simulink model "Demo919"  (R2018b)
settings: Solver=ode3  StartTime=0.0  StopTime=10  FixedStep=0.0005  RelTol=1e-3  EnableMultiTasking=on
values from neighbouring files (symbols this model uses):
  ADS1 = [1000 4000]    [data_new1.m]
  ADS2 = [900 4100]    [data_new1.m]
  br_opening = [0 20 40 60 80 100]    [data_new1.m]
  BRAKE = [485 1288 2091 2894 3697 4500]    [data_new1.m]
  InerWheel_Angle = [0 0.001 0.502 1.006 1.514 2.024 2.538 3.055 3.575 4.098 4.625 5.155 5.689 6.226 6.767 7.311 7.859 8.411 8.967 9.527 10.091 10.659 11.231 11.807 12.387 12.972 13.561 14.154 14.752 15.354 15.961 16.572 17.187 17.807 18.432 19.062 19.696 20.334 20.977 21.625 22.277 22.934 23.596 24.262 24.932 25.607 26.286 26.970 27.657 28.349 29.045 29.745 30.448 31.155 31.866]    [data_new1.m]
  OuterWheel_Angle = [0 0.001 0.501 1.001 1.501 2.001 2.501	3.001 3.501	4.001 4.501	5.001 5.501	6.001 6.501	7.001 7.501	8.001 8.501	9.001 9.501	10.001 10.501 11.001 11.501 12.001 12.501 13.001 13.501	14.001 14.501 15.001 15.501 16.001 16.501 17.001 17.501 18.001 18.501 19.001 19.501	20.001 20.501 21.001 21.501	22.001 22.501 23.001 23.501	24.001 24.501 25.001 25.501 26.001 26.501]    [data_new1.m]
  PUMP = [0 1000 2000 3000 4000 5000]    [data_new1.m]
  SteeringAngle_Cal = [-90 0 90]    [data_new1.m]
  SteeringAngle_Sensor = [640 1840 3041]    [data_new1.m]
  th_opening = [0 100]    [data_new1.m]
undefined symbols (not defined in the file or in its folder): D, I_AN06_5V, I_AN08_5V, I_AN09_5V, I_AN10_5V, I_HALL1, I_HALL2, I_SW01_L, I_SW10_L, I_SW11_H, I_SW12_H, I_SW13_H, I_SW14_H, I_SW15_H, I_SW16_H, I_SW17_H, I_SW18_H, I_SW19_H, I_SW20_H, O_PWM1_LS0A7, O_PWM2_LS0A7, O_SW02_LS0A4, O_SW13_HS1A, O_SW14_HS1A
libraries: ec5744lib x137, simulink x20, canmsglib x11
(part 1 of 5)
settings Model: Creator=30855  LastModifiedBy=Lenovo
settings OptimizationCC: DefaultParameterBehavior=Inlined  InlineInvariantSignals=on  EnhancedBackFolding=on  ExpressionFolding=off  PassReuseOutputArgsAs=Individual arguments  RollThreshold=65  StateBitsets=on  DataBitsets=on  ZeroExternalMemoryAtStartup=off  ZeroInternalMemoryAtStartup=off  EfficientFloat2IntCast=on  OptimizeBlockOrder=speed  DifferentSizesBufferReuse=on
settings DebuggingCC: InheritedTsInSrcMsg=none  ParameterTunabilityLossMsg=error
settings HardwareCC: ProdBitPerPointer=32  ProdBitPerSizeT=32  ProdBitPerPtrDiffT=32  ProdLargestAtomicInteger=Long  ProdLargestAtomicFloat=Double  ProdEndianess=BigEndian  ProdWordSize=32  ProdHWDeviceType=Freescale MPC5500
settings SFSimCC: MATLABDynamicMemAlloc=off
settings RTWCC: SystemTargetFile=ec5744.tlc  MakeCommand=make_rtw optimized_fixed_point=1  GenerateMakefile=off  TemplateMakefile=ec5744_lcc.tmf  PostCodeGenCommand=ec5744_pst_s2(buildInfo)  Description=Target for EC5744  GenerateReport=on  IncludeHyperlinkInReport=on  LaunchReport=on  GenerateTraceInfo=on  GenerateTraceReport=on  GenerateTraceReportSl=on  GenerateTraceReportSf=on  GenerateTraceReportEml=on
settings CodeAppCC: ForceParamTrailComments=on  IgnoreCustomStorageClasses=off  OperatorAnnotations=on  SimulinkDataObjDesc=on  SFDataObjDesc=on  InsertBlockDesc=on
settings STFCustomTargetCC: TargetLangStandard=C99 (ISO)  MultiwordLength=256  ModelReferenceCompliant=off  IncludeMdlTerminateFcn=off  CombineOutputUpdateFcns=on  SuppressErrorStatus=on  ERTCustomFileBanners=on  SupportContinuousTime=off  SupportNonInlinedSFcns=off  RemoveResetFunc=on  MATLABClassNameForMDSCustomization=Simulink.SoftwareTarget.ERTCustomization  SystemTargetFile=ec5744.tlc
settings ERTTargetCC: TargetLangStandard=C99 (ISO)  ModelReferenceCompliant=off  ParMdlRefBuildCompliant=off  CompOptLevelCompliant=off  ConcurrentExecutionCompliant=off  IncludeMdlTerminateFcn=off  SuppressErrorStatus=on  ModelStepFunctionPrototypeControlCompliant=off  CPPClassGenCompliant=off  UseToolchainInfoCompliant=off  GenerateASAP2=on  InlinedParameterPlacement=NonHierarchical  ERTSrcFileBannerTemplate=ec5744_code_template.cgt  ERTHdrFileBannerTemplate=ec5744_code_template.cgt  ERTDataSrcFileTemplate=ec5744_code_template.cgt  ERTDataHdrFileTemplate=ec5744_code_template.cgt  ERTCustomFileTemplate=ec5744_file_process.tlc

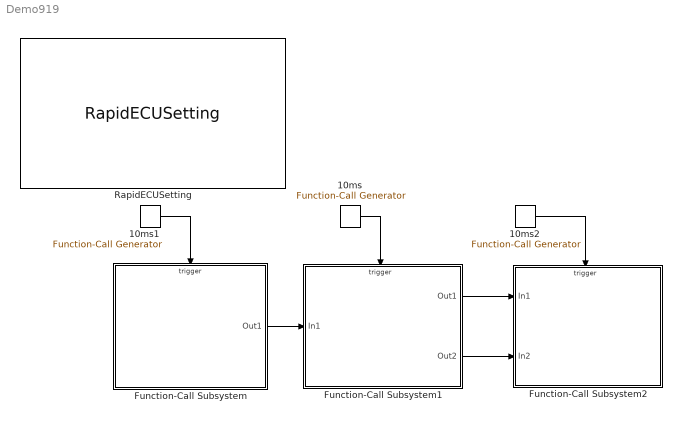
== system Demo919 ==
  10ms : simulink/Ports & Subsystems/Function-Call Generator  sample_time=0.01  numberOfIterations=1
  10ms1 : simulink/Ports & Subsystems/Function-Call Generator  sample_time=0.01  numberOfIterations=1
  10ms2 : simulink/Ports & Subsystems/Function-Call Generator  sample_time=0.01  numberOfIterations=1
  Function-Call Subsystem : Subsystem  TreatAsAtomicUnit=on
  Function-Call Subsystem1 : Subsystem  TreatAsAtomicUnit=on
  Function-Call Subsystem2 : Subsystem  TreatAsAtomicUnit=on
  RapidECUSetting : ec5744lib/RapidECU_U3/RapidECUSetting
      link override CAN: apdf=9  acmt=Extended(29-bit ID)  bpdf=9  cpdf=4  aboi=off  bcmt=Standard(11-bit ID)
      link override LIN: abrt=19200
      settings: SourceProductName=ECUCoder for MPC5744
  wires:
  10ms/1 -> Function-Call Subsystem1/Trigger
  Function-Call Subsystem/1(Out1) -> Function-Call Subsystem1/1(In1)
  Function-Call Subsystem1/1(Out1) -> Function-Call Subsystem2/1(In1)
  Function-Call Subsystem1/2(Out2) -> Function-Call Subsystem2/2(In2)
  10ms1/1 -> Function-Call Subsystem/Trigger
  10ms2/1 -> Function-Call Subsystem2/Trigger

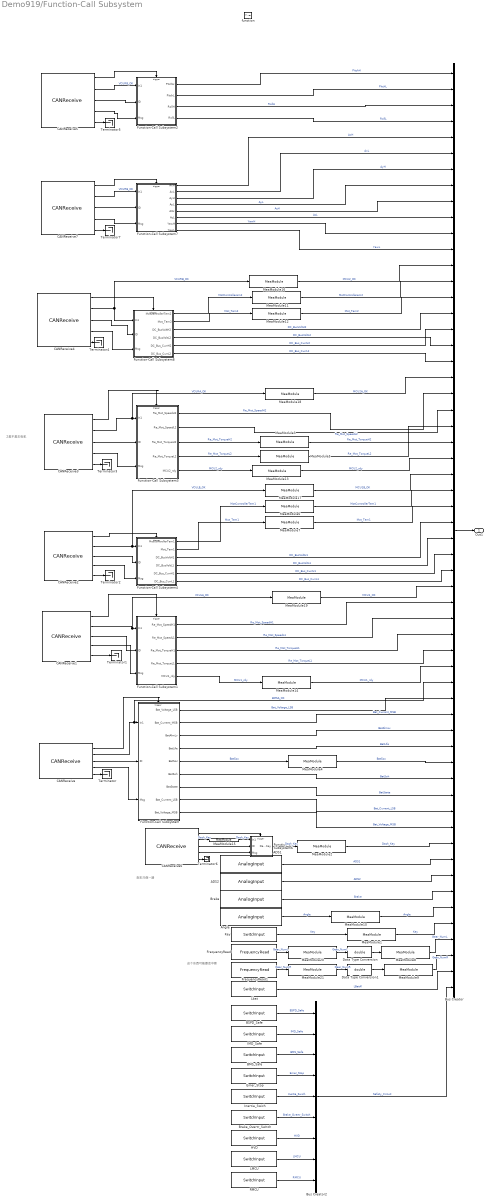
== system Demo919/Function-Call Subsystem ==
  note: 2是不是左电机
  note: 这个东西可能要走中断
  note: 刹车只做一路
  function : TriggerPort  TriggerType=function-call  VariantControl=Variant
  ADS1 : ec5744lib/RapidECU_U3/01BasicInput/AnalogInput  channel=54:I_AN08_5V  sampletime=-1
      settings: SourceProductName=ECUCoder for MPC5744
  ADS2 : ec5744lib/RapidECU_U3/01BasicInput/AnalogInput  channel=55:I_AN09_5V  sampletime=-1
      settings: SourceProductName=ECUCoder for MPC5744
  Angle : ec5744lib/RapidECU_U3/01BasicInput/AnalogInput  channel=56:I_AN10_5V  sampletime=-1
      settings: SourceProductName=ECUCoder for MPC5744
  BMS_Safe : ec5744lib/RapidECU_U3/01BasicInput/SwitchInput  channel=100:I_SW14_H  sampletime=-1
      settings: SourceProductName=ECUCoder for MPC5744
  BSPD_Safe : ec5744lib/RapidECU_U3/01BasicInput/SwitchInput  channel=46:I_SW12_H  sampletime=-1
      settings: SourceProductName=ECUCoder for MPC5744
  Brake : ec5744lib/RapidECU_U3/01BasicInput/AnalogInput  channel=52:I_AN06_5V  sampletime=-1
      settings: SourceProductName=ECUCoder for MPC5744
  Brake_Overtr_Switch : ec5744lib/RapidECU_U3/01BasicInput/SwitchInput  channel=104:I_SW17_H  sampletime=-1
      settings: SourceProductName=ECUCoder for MPC5744
  Bus Creator : BusCreator  Inputs=58
  Bus Creator2 : BusCreator  Inputs=9
  CANReceive : ec5744lib/RapidECU_U3/04CANCommunication/CANReceive  canmodule=0  canbuffer=16  canmessageid=hex2dec('186040F3')  canmessagetype=Extended(29-bit ID)  datalength=8  sampletime=-1
      settings: SourceProductName=ECUCoder for MPC5744
  CANReceive1 : ec5744lib/RapidECU_U3/04CANCommunication/CANReceive  canmodule=0  canbuffer=6  canmessageid=hex2dec('CFFC6EF')  canmessagetype=Extended(29-bit ID)  datalength=8  sampletime=-1
      settings: SourceProductName=ECUCoder for MPC5744
  CANReceive2 : ec5744lib/RapidECU_U3/04CANCommunication/CANReceive  canmodule=0  canbuffer=4  canmessageid=hex2dec('CFFC7EF')  canmessagetype=Extended(29-bit ID)  datalength=8  sampletime=-1
      settings: SourceProductName=ECUCoder for MPC5744
  CANReceive3 : ec5744lib/RapidECU_U3/04CANCommunication/CANReceive  canmodule=0  canbuffer=2  canmessageid=hex2dec('CB221EF')  canmessagetype=Extended(29-bit ID)  datalength=8  sampletime=-1
      settings: SourceProductName=ECUCoder for MPC5744
  CANReceive4 : ec5744lib/RapidECU_U3/04CANCommunication/CANReceive  canmodule=0  canbuffer=0  canmessageid=hex2dec('CB321EF')  canmessagetype=Extended(29-bit ID)  datalength=8  sampletime=-1
      settings: SourceProductName=ECUCoder for MPC5744
  CANReceive5 : ec5744lib/RapidECU_U3/04CANCommunication/CANReceive  canmodule=1  canbuffer=0  canmessageid=hex2dec('157')  canmessagetype=Standard(11-bit ID)  datalength=8  sampletime=-1
      settings: SourceProductName=ECUCoder for MPC5744
  CANReceive6 : ec5744lib/RapidECU_U3/04CANCommunication/CANReceive  canmodule=1  canbuffer=5  canmessageid=hex2dec('155')  canmessagetype=Standard(11-bit ID)  datalength=8  sampletime=-1
      settings: SourceProductName=ECUCoder for MPC5744
  CANReceive7 : ec5744lib/RapidECU_U3/04CANCommunication/CANReceive  canmodule=1  canbuffer=0  canmessageid=hex2dec('156')  canmessagetype=Standard(11-bit ID)  datalength=8  sampletime=-1
      settings: SourceProductName=ECUCoder for MPC5744
  Data Type Conversion : DataTypeConversion  OutDataTypeStr=double
  Data Type Conversion1 : DataTypeConversion  OutDataTypeStr=double
  Emer_Stop : ec5744lib/RapidECU_U3/01BasicInput/SwitchInput  channel=102:I_SW15_H  sampletime=-1
      settings: SourceProductName=ECUCoder for MPC5744
  FrequencyRead : ec5744lib/RapidECU_U3/01BasicInput/FrequencyRead  channel=37:I_HALL1  sampletime=-1
      settings: SourceProductName=ECUCoder for MPC5744
  FrequencyRead1 : ec5744lib/RapidECU_U3/01BasicInput/FrequencyRead  channel=103:I_SW16_H/I_HALL2  sampletime=-1
      settings: SourceProductName=ECUCoder for MPC5744
  Function-Call Subsystem : Subsystem  TreatAsAtomicUnit=on
  Function-Call Subsystem1 : Subsystem  TreatAsAtomicUnit=on
  Function-Call Subsystem2 : Subsystem  TreatAsAtomicUnit=on
  Function-Call Subsystem3 : Subsystem  TreatAsAtomicUnit=on
  Function-Call Subsystem4 : Subsystem  TreatAsAtomicUnit=on
  Function-Call Subsystem6 : Subsystem  TreatAsAtomicUnit=on
  Function-Call Subsystem7 : Subsystem  TreatAsAtomicUnit=on
  Function-Call Subsystem8 : Subsystem  TreatAsAtomicUnit=on
  HVD : ec5744lib/RapidECU_U3/01BasicInput/SwitchInput  channel=105:I_SW18_H  sampletime=-1
      settings: SourceProductName=ECUCoder for MPC5744
  IMD_Safe : ec5744lib/RapidECU_U3/01BasicInput/SwitchInput  channel=65:I_SW13_H  sampletime=-1
      settings: SourceProductName=ECUCoder for MPC5744
  Inertia_Swich : ec5744lib/RapidECU_U3/01BasicInput/SwitchInput  channel=44:I_SW11_H  sampletime=-1
      settings: SourceProductName=ECUCoder for MPC5744
  Key : ec5744lib/RapidECU_U3/01BasicInput/SwitchInput  channel=29:I_SW10_L  sampletime=-1
      settings: SourceProductName=ECUCoder for MPC5744
  LMCU : ec5744lib/RapidECU_U3/01BasicInput/SwitchInput  channel=112:I_SW19_H  sampletime=-1
      settings: SourceProductName=ECUCoder for MPC5744
  Lbat : ec5744lib/RapidECU_U3/01BasicInput/SwitchInput  channel=6:I_SW01_L  sampletime=-1
      settings: SourceProductName=ECUCoder for MPC5744
  MeaModule1 : ec5744lib/RapidECU_U3/07Calibration/MeaModule  signal=Key
      settings: SourceProductName=ECUCoder for MPC5744
  MeaModule10 : ec5744lib/RapidECU_U3/07Calibration/MeaModule  signal=Angle
      settings: SourceProductName=ECUCoder for MPC5744
  MeaModule11 : ec5744lib/RapidECU_U3/07Calibration/MeaModule  signal=MotConTem2
      settings: SourceProductName=ECUCoder for MPC5744
  MeaModule12 : ec5744lib/RapidECU_U3/07Calibration/MeaModule  signal=MotTem2
      settings: SourceProductName=ECUCoder for MPC5744
  MeaModule13 : ec5744lib/RapidECU_U3/07Calibration/MeaModule  signal=MCU2_rdy
      settings: SourceProductName=ECUCoder for MPC5744
  MeaModule14 : ec5744lib/RapidECU_U3/07Calibration/MeaModule  signal=MCU1_rdy
      settings: SourceProductName=ECUCoder for MPC5744
  MeaModule15 : ec5744lib/RapidECU_U3/07Calibration/MeaModule  signal=CANOK
      settings: SourceProductName=ECUCoder for MPC5744
  MeaModule16 : ec5744lib/RapidECU_U3/07Calibration/MeaModule  signal=MCU2B_OK
      settings: SourceProductName=ECUCoder for MPC5744
  MeaModule17 : ec5744lib/RapidECU_U3/07Calibration/MeaModule  signal=MCU1B_OK
      settings: SourceProductName=ECUCoder for MPC5744
  MeaModule18 : ec5744lib/RapidECU_U3/07Calibration/MeaModule  signal=MCU2A_OK
      settings: SourceProductName=ECUCoder for MPC5744
  MeaModule19 : ec5744lib/RapidECU_U3/07Calibration/MeaModule  signal=MCU1A_OK
      settings: SourceProductName=ECUCoder for MPC5744
  MeaModule2 : ec5744lib/RapidECU_U3/07Calibration/MeaModule  signal=Dash_KEY
      settings: SourceProductName=ECUCoder for MPC5744
  MeaModule20 : ec5744lib/RapidECU_U3/07Calibration/MeaModule  signal=HALL_l
      settings: SourceProductName=ECUCoder for MPC5744
  MeaModule21 : ec5744lib/RapidECU_U3/07Calibration/MeaModule  signal=HALL_r
      settings: SourceProductName=ECUCoder for MPC5744
  MeaModule3 : ec5744lib/RapidECU_U3/07Calibration/MeaModule  signal=Re_Mot_ToqH
      settings: SourceProductName=ECUCoder for MPC5744
  MeaModule4 : ec5744lib/RapidECU_U3/07Calibration/MeaModule  signal=BatSoc
      settings: SourceProductName=ECUCoder for MPC5744
  MeaModule5 : ec5744lib/RapidECU_U3/07Calibration/MeaModule  signal=Re_MotToqL
      settings: SourceProductName=ECUCoder for MPC5744
  MeaModule6 : ec5744lib/RapidECU_U3/07Calibration/MeaModule  signal=MotConTem1
      settings: SourceProductName=ECUCoder for MPC5744
  MeaModule7 : ec5744lib/RapidECU_U3/07Calibration/MeaModule  signal=MotTem1
      settings: SourceProductName=ECUCoder for MPC5744
  MeaModule8 : ec5744lib/RapidECU_U3/07Calibration/MeaModule  signal=HALL_L
      settings: SourceProductName=ECUCoder for MPC5744
  MeaModule9 : ec5744lib/RapidECU_U3/07Calibration/MeaModule  signal=HALL_R
      settings: SourceProductName=ECUCoder for MPC5744
  RMCU : ec5744lib/RapidECU_U3/01BasicInput/SwitchInput  channel=113:I_SW20_H  sampletime=-1
      settings: SourceProductName=ECUCoder for MPC5744
  Terminator{,1..7} (8 alike) : Terminator
  Out1 : Outport
  wires:
  ADS1/1 -> Bus Creator/50  "ADS1"
  ADS2/1 -> Bus Creator/51  "ADS2"
  Brake/1 -> Bus Creator/52  "Brake"
  Angle/1 -> MeaModule10/1  "Angle"
  Bus Creator/1 -> Out1/1
  Key/1 -> MeaModule1/1  "Key"
  CANReceive/1 -> Function-Call Subsystem/Trigger
  CANReceive/2 -> Bus Creator/39, Function-Call Subsystem/1(In1)  "BMSA_OK"
  CANReceive/3 -> Function-Call Subsystem/2(ID)
  CANReceive/4 -> Function-Call Subsystem/3(Msg)
  CANReceive/5 -> Terminator/1
  Function-Call Subsystem/1(Bat_Voltage_LSB) -> Bus Creator/40  "Bat_Voltage_LSB"
  Function-Call Subsystem/2(Bat_Current_MSB) -> Bus Creator/41  "Bat_Current_MSB"
  Function-Call Subsystem/3(BatAlmLv) -> Bus Creator/42  "BatAlmLv"
  Function-Call Subsystem/4(BatLife) -> Bus Creator/43  "BatLife"
  Function-Call Subsystem/5(BatSoc) -> MeaModule4/1  "BatSoc"
  Function-Call Subsystem/6(BatSoh) -> Bus Creator/45  "BatSoh"
  Function-Call Subsystem/7(BatState) -> Bus Creator/46  "BatState"
  Function-Call Subsystem/8(Bat_Current_LSB) -> Bus Creator/47  "Bat_Current_LSB"
  FrequencyRead/1 -> MeaModule20/1  "Gear_NumL"
  CANReceive1/5 -> Terminator1/1
  CANReceive1/4 -> Function-Call Subsystem1/3(Msg)
  CANReceive1/3 -> Function-Call Subsystem1/2(ID)
  CANReceive1/2 -> MeaModule19/1, Function-Call Subsystem1/1(In1)  "VCULA_OK"
  CANReceive1/1 -> Function-Call Subsystem1/Trigger
  CANReceive2/1 -> Function-Call Subsystem4/Trigger
  CANReceive2/2 -> Function-Call Subsystem4/1(In1), MeaModule17/1  "VCULB_OK"
  CANReceive2/3 -> Function-Call Subsystem4/2(ID)
  CANReceive2/4 -> Function-Call Subsystem4/3(Msg)
  CANReceive2/5 -> Terminator2/1
  CANReceive3/5 -> Terminator3/1
  CANReceive3/4 -> Function-Call Subsystem3/3(Msg)
  CANReceive3/3 -> Function-Call Subsystem3/2(ID)
  CANReceive3/2 -> MeaModule18/1, Function-Call Subsystem3/1(In1)  "VCURA_OK"
  CANReceive3/1 -> Function-Call Subsystem3/Trigger
  CANReceive4/1 -> Function-Call Subsystem8/Trigger
  CANReceive4/2 -> Function-Call Subsystem8/1(In1), MeaModule16/1  "VCURB_OK"
  CANReceive4/3 -> Function-Call Subsystem8/2(ID)
  CANReceive4/4 -> Function-Call Subsystem8/3(Msg)
  CANReceive4/5 -> Terminator4/1
  Function-Call Subsystem1/4(Re_Mot_TorqueL1) -> Bus Creator/37  "Re_Mot_TorqueL1"
  Function-Call Subsystem1/3(Re_Mot_TorqueH1) -> Bus Creator/36  "Re_Mot_TorqueH1"
  Function-Call Subsystem1/2(Re_Mot_SpeedL1) -> Bus Creator/35  "Re_Mot_SpeedL1"
  Function-Call Subsystem1/1(Re_Mot_SpeedH1) -> Bus Creator/34  "Re_Mot_SpeedH1"
  Function-Call Subsystem4/2(Mot_Tem1) -> MeaModule7/1  "Mot_Tem1"
  Function-Call Subsystem4/1(MotControllerTem1) -> MeaModule6/1  "MotControllerTem1"
  Function-Call Subsystem3/4(Re_Mot_TorqueL2) -> MeaModule5/1  "Re_Mot_TorqueL2"
  Function-Call Subsystem3/3(Re_Mot_TorqueH2) -> MeaModule3/1  "Re_Mot_TorqueH2"
  Function-Call Subsystem3/2(Re_Mot_SpeedL2) -> Bus Creator/22  "Re_Mot_SpeedL2"
  Function-Call Subsystem3/1(Re_Mot_SpeedH2) -> Bus Creator/21  "Re_Mot_SpeedH2"
  Function-Call Subsystem8/2(Mot_Tem2) -> MeaModule12/1  "Mot_Tem2"
  Function-Call Subsystem8/1(MotControllerTem2) -> MeaModule11/1  "MotControllerem2"
  Function-Call Subsystem/9(Bat_Voltage_MSB) -> Bus Creator/48  "Bat_Voltage_MSB"
  FrequencyRead1/1 -> MeaModule21/1  "Gear_NumR"
  CANReceive6/1 -> Function-Call Subsystem6/Trigger
  CANReceive6/3 -> Function-Call Subsystem6/2(ID)
  CANReceive6/4 -> Function-Call Subsystem6/3(Msg)
  CANReceive6/5 -> Terminator6/1
  Function-Call Subsystem6/1(Dash_Key) -> MeaModule2/1  "Dash_Key"
  MeaModule1/1 -> Bus Creator/54  "Key"
  MeaModule3/1 -> Bus Creator/23  "Re_Mot_TorqueH2"
  MeaModule5/1 -> Bus Creator/24  "Re_Mot_TorqueL2"
  MeaModule6/1 -> Bus Creator/27  "MotControllerTem1"
  MeaModule7/1 -> Bus Creator/28  "Mot_Tem1"
  MeaModule8/1 -> Bus Creator/55  "Gear_NumL"
  MeaModule9/1 -> Bus Creator/56  "Gear_NumR"
  MeaModule11/1 -> Bus Creator/14  "MotControllerem2"
  MeaModule12/1 -> Bus Creator/15  "Mot_Tem2"
  MeaModule2/1 -> Bus Creator/49  "Dash_Key"
  CANReceive6/2 -> MeaModule15/1  "Dash_Key"
  Function-Call Subsystem4/3(DC_BusVoltH1) -> Bus Creator/29  "DC_BusVoltH1"
  Function-Call Subsystem8/3(DC_BusVoltH2) -> Bus Creator/16  "DC_BusVoltH2"
  Function-Call Subsystem8/6("DC_Bus_CurrL2 ") -> Bus Creator/19  "DC_Bus_CurrL2"
  Function-Call Subsystem4/4(DC_BusVoltL1) -> Bus Creator/30  "DC_BusVoltL1"
  MeaModule4/1 -> Bus Creator/44  "BatSoc"
  Function-Call Subsystem1/5(MCU1_rdy) -> MeaModule14/1  "MCU1_rdy"
  Function-Call Subsystem3/5(MCU2_rdy) -> MeaModule13/1  "MCU2_rdy"
  Data Type Conversion/1 -> MeaModule8/1
  Data Type Conversion1/1 -> MeaModule9/1
  CANReceive7/1 -> Function-Call Subsystem7/Trigger
  CANReceive7/3 -> Function-Call Subsystem7/2(ID)
  CANReceive7/4 -> Function-Call Subsystem7/3(Msg)
  CANReceive7/2 -> Function-Call Subsystem7/1(In1)  "VCURB_OK"
  CANReceive7/5 -> Terminator7/1
  Function-Call Subsystem7/1(AxH) -> Bus Creator/5  "AxH"
  Function-Call Subsystem7/8(YawL) -> Bus Creator/12  "YawL"
  Function-Call Subsystem7/7(YawH) -> Bus Creator/11  "YawH"
  Function-Call Subsystem7/6(AzL) -> Bus Creator/10  "AzL"
  Function-Call Subsystem7/5(AzH) -> Bus Creator/9  "AzH"
  Function-Call Subsystem7/4(AyL) -> Bus Creator/8  "AyL"
  Function-Call Subsystem7/3(AyH) -> Bus Creator/7  "AyH"
  MeaModule10/1 -> Bus Creator/53  "Angle"
  MeaModule13/1 -> Bus Creator/25  "MCU2_rdy"
  MeaModule14/1 -> Bus Creator/38  "MCU1_rdy"
  Function-Call Subsystem7/2(AxL) -> Bus Creator/6  "AxL"
  MeaModule15/1 -> Function-Call Subsystem6/1(In1)  "Dash_Key"
  Function-Call Subsystem8/4(DC_BusVoltL2) -> Bus Creator/18  "DC_BusVoltL2"
  Function-Call Subsystem8/5(DC_Bus_CurrH2) -> Bus Creator/17  "DC_Bus_CurrH2"
  Function-Call Subsystem4/5(DC_Bus_CurrH1) -> Bus Creator/31  "DC_Bus_CurrH1"
  Function-Call Subsystem4/6(DC_Bus_CurrL1) -> Bus Creator/32  "DC_Bus_CurrL1"
  MeaModule16/1 -> Bus Creator/13  "MCU2_OK"
  MeaModule18/1 -> Bus Creator/20  "MCU2A_OK"
  MeaModule17/1 -> Bus Creator/26  "MCU1B_OK"
  MeaModule19/1 -> Bus Creator/33  "MCU1_OK"
  CANReceive5/2 -> Function-Call Subsystem2/1(In1)  "VCURB_OK"
  CANReceive5/4 -> Function-Call Subsystem2/3(Msg)
  CANReceive5/3 -> Function-Call Subsystem2/2(ID)
  CANReceive5/5 -> Terminator5/1
  CANReceive5/1 -> Function-Call Subsystem2/Trigger
  Function-Call Subsystem2/1(PitchH) -> Bus Creator/1  "PitchH"
  Function-Call Subsystem2/2(PitchL) -> Bus Creator/2  "PitchL"
  Function-Call Subsystem2/3(RollH) -> Bus Creator/3  "RollH"
  Function-Call Subsystem2/4(RollL) -> Bus Creator/4  "RollL"
  Lbat/1 -> Bus Creator/57  "LBatAl"
  Bus Creator2/1 -> Bus Creator/58  "Safety_Circuit"
  HVD/1 -> Bus Creator2/7  "HVD"
  Inertia_Swich/1 -> Bus Creator2/5  "Inertia_Swich"
  BSPD_Safe/1 -> Bus Creator2/1  "BSPD_Safe"
  RMCU/1 -> Bus Creator2/9  "RMCU"
  Emer_Stop/1 -> Bus Creator2/4  "Emer_Stop"
  Brake_Overtr_Switch/1 -> Bus Creator2/6  "Brake_Overtr_Switch"
  LMCU/1 -> Bus Creator2/8  "LMCU"
  BMS_Safe/1 -> Bus Creator2/3  "BMS_Safe"
  IMD_Safe/1 -> Bus Creator2/2  "IMD_Safe"
  MeaModule20/1 -> Data Type Conversion/1  "Gear_NumL"
  MeaModule21/1 -> Data Type Conversion1/1  "Gear_NumR"

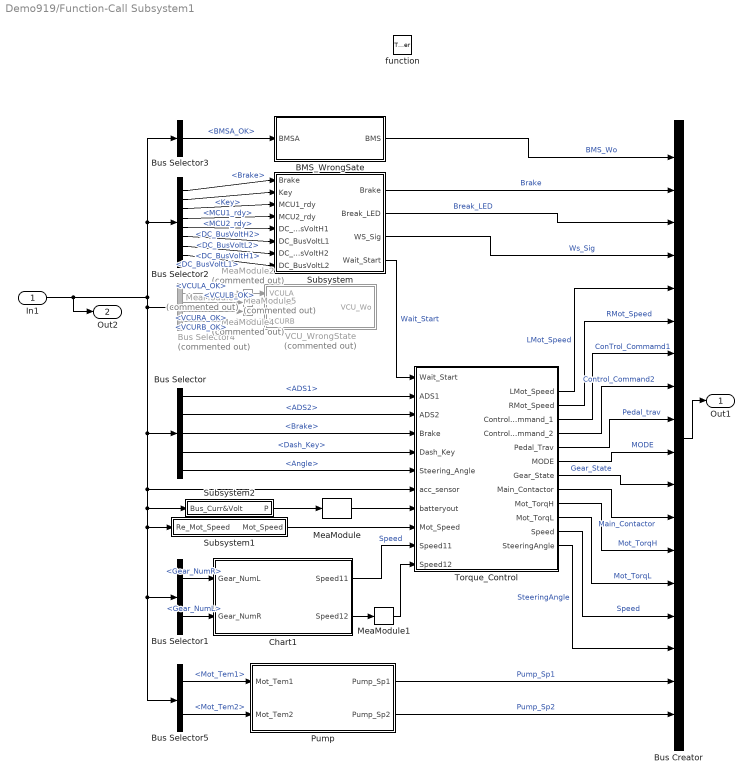
== system Demo919/Function-Call Subsystem1 ==
  In1 : Inport
  "  function" : TriggerPort  TriggerType=function-call  VariantControl=Variant
  BMS_WrongSate : Stateflow chart  TreatAsAtomicUnit=on
  Bus Creator : BusCreator  Inputs=18
  Bus Selector : BusSelector  OutputSignals=ADS1,ADS2,Brake,Dash_Key,Angle
  Bus Selector1 : BusSelector  OutputSignals=Gear_NumR,Gear_NumL
  Bus Selector2 : BusSelector  OutputSignals=Brake,Key,MCU1_rdy,MCU2_rdy,DC_BusVoltH2,DC_BusVoltL2,DC_BusVoltH1,DC_BusVoltL1
  Bus Selector3 : BusSelector  OutputSignals=BMSA_OK
  Bus Selector4 : BusSelector  Commented=on  OutputSignals=VCULA_OK,VCULB_OK,VCURA_OK,VCURB_OK
  Bus Selector5 : BusSelector  OutputSignals=Mot_Tem1,Mot_Tem2
  Chart1 : Stateflow chart  TreatAsAtomicUnit=on
  MeaModule : ec5744lib/RapidECU_U3/07Calibration/MeaModule  signal=P
      settings: SourceProductName=ECUCoder for MPC5744
  MeaModule1 : ec5744lib/RapidECU_U3/07Calibration/MeaModule  signal=S12
      settings: SourceProductName=ECUCoder for MPC5744
  MeaModule2 : ec5744lib/RapidECU_U3/07Calibration/MeaModule  Commented=on  signal=VCULA
      settings: SourceProductName=ECUCoder for MPC5744
  MeaModule3 : ec5744lib/RapidECU_U3/07Calibration/MeaModule  Commented=on  signal=VCUlb
      settings: SourceProductName=ECUCoder for MPC5744
  MeaModule4 : ec5744lib/RapidECU_U3/07Calibration/MeaModule  Commented=on  signal=VCUra
      settings: SourceProductName=ECUCoder for MPC5744
  MeaModule5 : ec5744lib/RapidECU_U3/07Calibration/MeaModule  Commented=on  signal=VCUrb
      settings: SourceProductName=ECUCoder for MPC5744
  Pump : Subsystem
  Subsystem : Subsystem
  Subsystem1 : Subsystem
  Subsystem2 : Subsystem
  Torque_Control : Subsystem
  VCU_WrongState : Stateflow chart  Commented=on  TreatAsAtomicUnit=on
  Out1 : Outport
  Out2 : Outport  Port=2
  wires:
  Bus Selector/1 -> Torque_Control/2(ADS1)  "<ADS1>"
  Bus Selector/2 -> Torque_Control/3(ADS2)  "<ADS2>"
  Torque_Control/1(LMot_Speed) -> Bus Creator/5  "LMot_Speed"
  Torque_Control/2(RMot_Speed) -> Bus Creator/6  "RMot_Speed"
  Bus Creator/1 -> Out1/1
  Bus Selector2/2 -> Subsystem/2(Key)  "<Key>"
  Subsystem/4(Wait_Start) -> Torque_Control/1(Wait_Start)  "Wait_Start"
  BMS_WrongSate/1(BMS) -> Bus Creator/1  "BMS_Wo"
  Torque_Control/3("Control_Command_1 ") -> Bus Creator/7  "ConTrol_Commamd1"
  Torque_Control/4(Control_Command_2) -> Bus Creator/8  "Control_Command2"
  Bus Selector2/1 -> Subsystem/1(Brake)  "<Brake>"
  Torque_Control/5(Pedal_Trav) -> Bus Creator/9  "Pedal_trav"
  Bus Selector/4 -> Torque_Control/5("Dash_Key ")  "<Dash_Key>"
  Bus Selector5/1 -> Pump/1(Mot_Tem1)  "<Mot_Tem1>"
  Bus Selector5/2 -> Pump/2(Mot_Tem2)  "<Mot_Tem2>"
  Pump/1(Pump_Sp1) -> Bus Creator/17  "Pump_Sp1"
  Pump/2(Pump_Sp2) -> Bus Creator/18  "Pump_Sp2"
  Subsystem/2(Break_LED) -> Bus Creator/3  "Break_LED"
  Bus Selector/3 -> Torque_Control/4("Brake ")  "<Brake>"
  Bus Selector3/1 -> BMS_WrongSate/1(BMSA)  "<BMSA_OK>"
  Bus Selector4/1 -> MeaModule2/1  "<VCULA_OK>"
  Bus Selector4/2 -> MeaModule3/1  "<VCULB_OK>"
  Bus Selector4/3 -> MeaModule4/1  "<VCURA_OK>"
  Bus Selector4/4 -> MeaModule5/1  "<VCURB_OK>"
  MeaModule2/1 -> VCU_WrongState/1(VCULA)
  MeaModule3/1 -> VCU_WrongState/2(VCULB)
  MeaModule4/1 -> VCU_WrongState/3(VCURA)
  MeaModule5/1 -> VCU_WrongState/4(VCURB)
  Bus Selector1/2 -> Chart1/2(Gear_NumR)  "<Gear_NumL>"
  Bus Selector1/1 -> Chart1/1(Gear_NumL)  "<Gear_NumR>"
  In1/1 -> Out2/1, Bus Selector4/1, Bus Selector5/1, Bus Selector1/1, Subsystem1/1(Re_Mot_Speed), Subsystem2/1(Bus_Curr&Volt), Torque_Control/7(acc_sensor), Bus Selector/1, Bus Selector3/1, Bus Selector2/1
  Torque_Control/11(Speed) -> Bus Creator/15  "Speed"
  Torque_Control/6(MODE) -> Bus Creator/10  "MODE"
  Subsystem/3(WS_Sig) -> Bus Creator/4  "Ws_Sig"
  Torque_Control/7("Gear_State ") -> Bus Creator/11  "Gear_State"
  Torque_Control/8(Main_Contactor) -> Bus Creator/12  "Main_Contactor"
  Bus Selector2/3 -> Subsystem/3(MCU1_rdy)  "<MCU1_rdy>"
  Bus Selector2/4 -> Subsystem/4(MCU2_rdy)  "<MCU2_rdy>"
  Bus Selector2/5 -> Subsystem/5(DC_BusVoltH1)  "<DC_BusVoltH2>"
  Bus Selector2/6 -> Subsystem/6(DC_BusVoltL1)  "<DC_BusVoltL2>"
  Bus Selector2/7 -> Subsystem/7(DC_BusVoltH2)  "<DC_BusVoltH1>"
  Bus Selector2/8 -> Subsystem/8(DC_BusVoltL2)  "<DC_BusVoltL1>"
  Subsystem/1("Brake ") -> Bus Creator/2  "Brake"
  Bus Selector/5 -> Torque_Control/6(Steering_Angle)  "<Angle>"
  Subsystem2/1(P) -> MeaModule/1
  Subsystem1/1(Mot_Speed) -> Torque_Control/9(Mot_Speed)
  Torque_Control/9(Mot_TorqH) -> Bus Creator/13  "Mot_TorqH"
  Torque_Control/10(Mot_TorqL) -> Bus Creator/14  "Mot_TorqL"
  Chart1/1(Speed11) -> Torque_Control/10(Speed11)  "Speed"
  Chart1/2(Speed12) -> MeaModule1/1
  MeaModule/1 -> Torque_Control/8(batteryout)
  MeaModule1/1 -> Torque_Control/11(Speed12)
  Torque_Control/12(SteeringAngle) -> Bus Creator/16  "SteeringAngle"

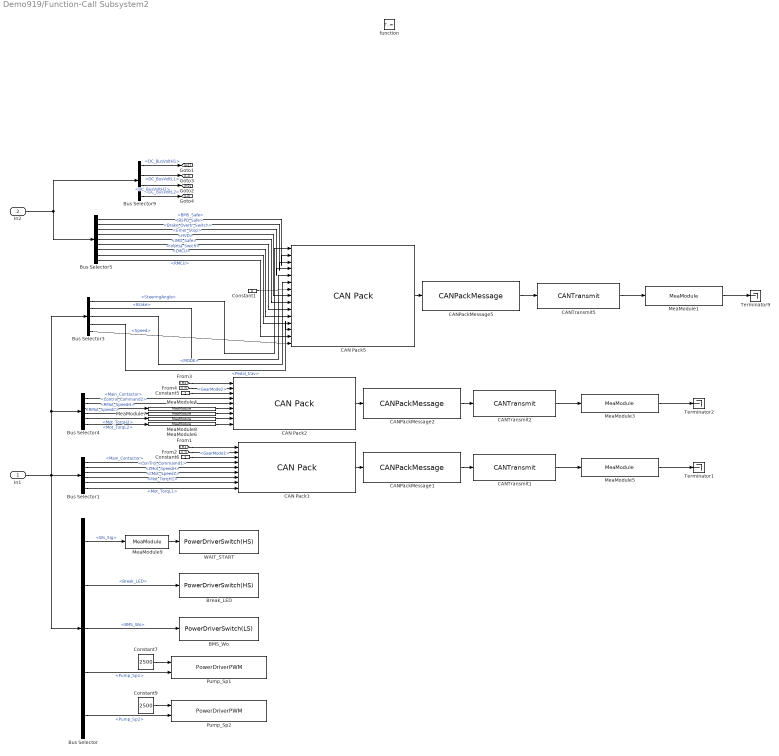
== system Demo919/Function-Call Subsystem2 ==
  In1 : Inport
  In2 : Inport  Port=2
  function : TriggerPort  TriggerType=function-call  VariantControl=Variant
  BMS_Wo : ec5744lib/RapidECU_U3/02PowerDriverSwitch/PowerDriverSwitch(LS)  channel=59:O_SW02_LS0A4  sampletime=-1
      settings: SourceProductName=ECUCoder for MPC5744
  Break_LED : ec5744lib/RapidECU_U3/02PowerDriverSwitch/PowerDriverSwitch(HS)  channel=115:O_SW13_HS1A  sampletime=-1
      settings: SourceProductName=ECUCoder for MPC5744
  Bus Selector : BusSelector  OutputSignals=Ws_Sig,Break_LED,BMS_Wo,Pump_Sp1,Pump_Sp2
  Bus Selector1 : BusSelector  OutputSignals=Main_Contactor,ConTrol_Commamd1,LMot_Speed.LMot_SpeedH,LMot_Speed.LMot_SpeedL,Mot_TorqH.Mot_TorqH1,Mot_TorqL.Mot_TorqL1
  Bus Selector3 : BusSelector  OutputSignals=SteeringAngle,Brake,MODE,Pedal_trav,Speed
  Bus Selector4 : BusSelector  OutputSignals=Main_Contactor,Control_Command2,RMot_Speed.RMot_SpeedH,RMot_Speed.RMot_SpeedL,Mot_TorqH.Mot_TorqH2,Mot_TorqL.Mot_TorqL2
  Bus Selector5 : BusSelector  OutputSignals=Safety_Circuit.BMS_Safe,Safety_Circuit.BSPD_Safe,Safety_Circuit.Brake_Overtr_Switch,Safety_Circuit.Emer_Stop,Safety_Circuit.HVD,Safety_Circuit.IMD_Safe,Safety_Circuit.Inertia_Swich,Safety_Circuit.LMCU,Safety_Circuit.RMCU
  Bus Selector9 : BusSelector  OutputSignals=DC_BusVoltH1,DC_BusVoltL1,DC_BusVoltH2,DC_BusVoltL2
  CAN Pack1 : canmsglib/CAN Pack  CANdbFile=E:\project\DBC_file\MotControl.dbc  MsgList=VCUtoMUC1  MsgName=VCUtoMUC1  MsgIDType=Extended (29-bit identifier)  MsgIdentifier=146927393  MsgLength=8  SignalInfo=DC_Bus_VoltageH1$48$8$1$2$1$0$1$0$0$255$#DC_Bus_VoltageL1$56$8$1$2$1$0$1$0$0$255$#GearState1$40$2$1$2$1$0$1$0$0$3$#Main_contactor1$43$1$1$2$1$0$1$0$0$1$#Tr_ControlMode_Command1$32$8$1$2$1$0$1$0$0$255$#Tr_Mot_SpeedH1$8$8$1$2$1$0$1$0$0$255$#Tr_Mot_SpeedL1$0$8$1$2$1$0$1$0$0$255$#Tr_Mot_TorqH1$24$8$1$2$1$0$1$0$0$255$#Tr_Mot_TorqL1$16$8$1$2$1$0$1$0$0$255$#  NSignals=9  StartBits=str2num('[int32(48);int32(56);int32(40);int32(43);int32(32);int32(8);int32(0);int32(24);int32(16)]')  SignalSizes=str2num('[int32(8);int32(8);int32(2);int32(1);int32(8);int32(8);int32(8);int32(8);int32(8)]')  ByteOrders=str2num('[int32(1);int32(1);int32(1);int32(1);int32(1);int32(1);int32(1);int32(1);int32(1)]')  DataTypes=str2num('[int32(2);int32(2);int32(2);int32(2);int32(2);int32(2);int32(2);int32(2);int32(2)]')  MultiplexTypes=str2num('[int32(1);int32(1);int32(1);int32(1);int32(1);int32(1);int32(1);int32(1);int32(1)]')  MultiplexValues=str2num('[double(0);double(0);double(0);double(0);double(0);double(0);double(0);double(0);double(0)]')  Factors=str2num('[double(1);double(1);double(1);double(1);double(1);double(1);double(1);double(1);double(1)]')  Offsets=str2num('[double(0);double(0);double(0);double(0);double(0);double(0);double(0);double(0);double(0)]')  Minimums=str2num('[double(0);double(0);double(0);double(0);double(0);double(0);double(0);double(0);double(0)]')  Maximums=str2num('[double(255);double(255);double(3);double(1);double(255);double(255);double(255);double(255);double(255)]')  Remote=off  ApplyMinMax=off  BusOutput=off
      settings: SourceProductName=Simulink Real-Time  SourceProductBaseCode=XP  DataFormat=CANdb specified signals
  CAN Pack2 : canmsglib/CAN Pack  CANdbFile=E:\project\DBC_file\MotControl.dbc  MsgList=VCUtoMCU2  MsgName=VCUtoMCU2  MsgIDType=Extended (29-bit identifier)  MsgIdentifier=145878817  MsgLength=8  SignalInfo=DC_Bus_VoltageH2$48$8$1$2$1$0$1$0$0$255$#DC_Bus_VoltrageL2$56$8$1$2$1$0$1$0$0$255$#GearState2$40$2$1$2$1$0$1$0$0$3$#Main_contactor2$43$1$1$2$1$0$1$0$0$1$#Tr_ControlMode_Command2$32$8$1$2$1$0$1$0$0$255$#Tr_Mot_SpeedH2$8$8$1$2$1$0$1$0$0$255$#Tr_Mot_SpeedL2$0$8$1$2$1$0$1$0$0$255$#Tr_Mot_TorqH2$24$8$1$2$1$0$1$0$0$255$#Tr_Mot_TorqL2$16$8$1$2$1$0$1$0$0$255$#  NSignals=9  StartBits=str2num('[int32(48);int32(56);int32(40);int32(43);int32(32);int32(8);int32(0);int32(24);int32(16)]')  SignalSizes=str2num('[int32(8);int32(8);int32(2);int32(1);int32(8);int32(8);int32(8);int32(8);int32(8)]')  ByteOrders=str2num('[int32(1);int32(1);int32(1);int32(1);int32(1);int32(1);int32(1);int32(1);int32(1)]')  DataTypes=str2num('[int32(2);int32(2);int32(2);int32(2);int32(2);int32(2);int32(2);int32(2);int32(2)]')  MultiplexTypes=str2num('[int32(1);int32(1);int32(1);int32(1);int32(1);int32(1);int32(1);int32(1);int32(1)]')  MultiplexValues=str2num('[double(0);double(0);double(0);double(0);double(0);double(0);double(0);double(0);double(0)]')  Factors=str2num('[double(1);double(1);double(1);double(1);double(1);double(1);double(1);double(1);double(1)]')  Offsets=str2num('[double(0);double(0);double(0);double(0);double(0);double(0);double(0);double(0);double(0)]')  Minimums=str2num('[double(0);double(0);double(0);double(0);double(0);double(0);double(0);double(0);double(0)]')  Maximums=str2num('[double(255);double(255);double(3);double(1);double(255);double(255);double(255);double(255);double(255)]')  Remote=off  ApplyMinMax=off  BusOutput=off
      settings: SourceProductName=Simulink Real-Time  SourceProductBaseCode=XP  DataFormat=CANdb specified signals
  CAN Pack5 : canmsglib/CAN Pack  CANdbFile=E:\project\DBC_file\MotControl.dbc  MsgList=VCUtoDash1  MsgName=VCUtoDash1  MsgIDType=Extended (29-bit identifier)  MsgIdentifier=529  MsgLength=8  SignalInfo=Angle$48$8$1$2$1$0$1$0$0$255$#BMS_Safe$33$1$1$2$1$0$1$0$0$1$#BSPD_Safe$40$1$1$2$1$0$1$0$0$1$#Brake_Overtr_Switch$36$1$1$2$1$0$1$0$0$1$#Brake_Val$16$8$1$2$1$0$1$0$0$255$#CarMode$45$3$1$2$1$0$1$0$0$7$#Distance$24$8$1$2$1$0$1$0$0$255$#Emer_Stop$34$1$1$2$1$0$1$0$0$1$#HVD$37$1$1$2$1$0$1$0$0$1$#IMD_Safe$32$1$1$2$1$0$1$0$0$1$#Inertia_Swich$35$1$1$2$1$0$1$0$0$1$#LMCU$38$1$1$2$1$0$1$0$0$1$#Ped_Trav$8$8$1$2$1$0$1$0$0$255$#RMCU$39$1$1$2$1$0$1$0$0$1$#Veh_Sp$0$8$1$2$1$0$1$0$0$255$#  NSignals=15  StartBits=str2num('[int32(48);int32(33);int32(40);int32(36);int32(16);int32(45);int32(24);int32(34);int32(37);int32(32);int32(35);int32(38);int32(8);int32(39);int32(0)]')  SignalSizes=str2num('[int32(8);int32(1);int32(1);int32(1);int32(8);int32(3);int32(8);int32(1);int32(1);int32(1);int32(1);int32(1);int32(8);int32(1);int32(8)]')  ByteOrders=str2num('[int32(1);int32(1);int32(1);int32(1);int32(1);int32(1);int32(1);int32(1);int32(1);int32(1);int32(1);int32(1);int32(1);int32(1);int32(1)]')  DataTypes=str2num('[int32(2);int32(2);int32(2);int32(2);int32(2);int32(2);int32(2);int32(2);int32(2);int32(2);int32(2);int32(2);int32(2);int32(2);int32(2)]')  MultiplexTypes=str2num('[int32(1);int32(1);int32(1);int32(1);int32(1);int32(1);int32(1);int32(1);int32(1);int32(1);int32(1);int32(1);int32(1);int32(1);int32(1)]')  MultiplexValues=str2num('[double(0);double(0);double(0);double(0);double(0);double(0);double(0);double(0);double(0);double(0);double(0);double(0);double(0);double(0);double(0)]')  Factors=str2num('[double(1);double(1);double(1);double(1);double(1);double(1);double(1);double(1);double(1);double(1);double(1);double(1);double(1);double(1);double(1)]')  Offsets=str2num('[double(0);double(0);double(0);double(0);double(0);double(0);double(0);double(0);double(0);double(0);double(0);double(0);double(0);double(0);double(0)]')  Minimums=str2num('[double(0);double(0);double(0);double(0);double(0);double(0);double(0);double(0);double(0);double(0);double(0);double(0);double(0);double(0);double(0)]')  Maximums=str2num('[double(255);double(1);double(1);double(1);double(255);double(7);double(255);double(1);double(1);double(1);double(1);double(1);double(255);double(1);double(255)]')  Remote=off  ApplyMinMax=off  BusOutput=off
      settings: SourceProductName=Simulink Real-Time  SourceProductBaseCode=XP  DataFormat=CANdb specified signals
  CANPackMessage1 : ec5744lib/RapidECU_U3/04CANCommunication/CANPackMessage  datalength=8  sampletime=-1
      settings: SourceProductName=ECUCoder for MPC5744
  CANPackMessage2 : ec5744lib/RapidECU_U3/04CANCommunication/CANPackMessage  datalength=8  sampletime=-1
      settings: SourceProductName=ECUCoder for MPC5744
  CANPackMessage5 : ec5744lib/RapidECU_U3/04CANCommunication/CANPackMessage  datalength=8  sampletime=-1
      settings: SourceProductName=ECUCoder for MPC5744
  CANTransmit1 : ec5744lib/RapidECU_U3/04CANCommunication/CANTransmit  canmodule=0  canbuffer=12  canmessageid=hex2dec('8C1EF21')  canmessagetype=Extended(29-bit ID)  datalength=8  sampletime=-1
      settings: SourceProductName=ECUCoder for MPC5744
  CANTransmit2 : ec5744lib/RapidECU_U3/04CANCommunication/CANTransmit  canmodule=0  canbuffer=10  canmessageid=hex2dec('8B1EF21')  canmessagetype=Extended(29-bit ID)  datalength=8  sampletime=-1
      settings: SourceProductName=ECUCoder for MPC5744
  CANTransmit5 : ec5744lib/RapidECU_U3/04CANCommunication/CANTransmit  canmodule=0  canbuffer=8  canmessageid=hex2dec('211')  canmessagetype=Extended(29-bit ID)  datalength=8  sampletime=-1
      settings: SourceProductName=ECUCoder for MPC5744
  Constant1 : Constant  Value=0
  Constant5 : Constant  Value=2
  Constant6 : Constant  Value=2
  Constant7 : Constant  Value=2500  OutDataTypeStr=uint16
  Constant9 : Constant  Value=2500  OutDataTypeStr=uint16
  MeaModule1 : ec5744lib/RapidECU_U3/07Calibration/MeaModule  signal=Dash1
      settings: SourceProductName=ECUCoder for MPC5744
  MeaModule3 : ec5744lib/RapidECU_U3/07Calibration/MeaModule  signal=VCUtoMCU2
      settings: SourceProductName=ECUCoder for MPC5744
  MeaModule4 : ec5744lib/RapidECU_U3/07Calibration/MeaModule  signal=SpeedH
      settings: SourceProductName=ECUCoder for MPC5744
  MeaModule5 : ec5744lib/RapidECU_U3/07Calibration/MeaModule  signal=VCUtoMCU
      settings: SourceProductName=ECUCoder for MPC5744
  MeaModule6 : ec5744lib/RapidECU_U3/07Calibration/MeaModule  signal=TorqL
      settings: SourceProductName=ECUCoder for MPC5744
  MeaModule7 : ec5744lib/RapidECU_U3/07Calibration/MeaModule  signal=SpeedL
      settings: SourceProductName=ECUCoder for MPC5744
  MeaModule8 : ec5744lib/RapidECU_U3/07Calibration/MeaModule  signal=TorqH
      settings: SourceProductName=ECUCoder for MPC5744
  MeaModule9 : ec5744lib/RapidECU_U3/07Calibration/MeaModule  signal=Ws_Sig
      settings: SourceProductName=ECUCoder for MPC5744
  Pump_Sp1 : ec5744lib/RapidECU_U3/03PowerDriverPWM/PowerDriverPWM  channel=60:O_PWM1_LS0A7  sampletime=-1
      settings: SourceProductName=ECUCoder for MPC5744
  Pump_Sp2 : ec5744lib/RapidECU_U3/03PowerDriverPWM/PowerDriverPWM  channel=90:O_PWM2_LS0A7  sampletime=-1
      settings: SourceProductName=ECUCoder for MPC5744
  Terminator1 : Terminator
  Terminator2 : Terminator
  Terminator9 : Terminator
  WAIT_START : ec5744lib/RapidECU_U3/02PowerDriverSwitch/PowerDriverSwitch(HS)  channel=117:O_SW14_HS1A  sampletime=-1
      settings: SourceProductName=ECUCoder for MPC5744
  wires:
  CANPackMessage1/1 -> CANTransmit1/1
  CANTransmit1/1 -> MeaModule5/1
  Bus Selector/1 -> MeaModule9/1  "<Ws_Sig>"
  CANTransmit2/1 -> MeaModule3/1
  CANPackMessage2/1 -> CANTransmit2/1
  Bus Selector4/5 -> MeaModule8/1  "<Mot_TorqH2>"
  Bus Selector4/6 -> MeaModule6/1  "<Mot_TorqL2>"
  Bus Selector4/3 -> MeaModule4/1  "<RMot_SpeedH>"
  Bus Selector4/4 -> MeaModule7/1  "<RMot_SpeedL>"
  Constant5/1 -> CAN Pack2/3  "<GearMode2>"
  Constant6/1 -> CAN Pack1/3  "<GearMode1>"
  Bus Selector1/2 -> CAN Pack1/5  "<ConTrol_Commamd1>"
  Bus Selector1/4 -> CAN Pack1/7  "<LMot_SpeedL>"
  Bus Selector1/3 -> CAN Pack1/6  "<LMot_SpeedH>"
  Bus Selector1/6 -> CAN Pack1/9  "<Mot_TorqL1>"
  Bus Selector1/5 -> CAN Pack1/8  "<Mot_TorqH1>"
  In1/1 -> Bus Selector/1, Bus Selector1/1, Bus Selector3/1, Bus Selector4/1
  MeaModule3/1 -> Terminator2/1
  MeaModule5/1 -> Terminator1/1
  Bus Selector/4 -> Pump_Sp1/2  "<Pump_Sp1>"
  Bus Selector/5 -> Pump_Sp2/2  "<Pump_Sp2>"
  Bus Selector/2 -> Break_LED/1  "<Break_LED>"
  Constant7/1 -> Pump_Sp1/1
  Constant9/1 -> Pump_Sp2/1
  Bus Selector4/2 -> CAN Pack2/5  "<Control_Command2>"
  MeaModule4/1 -> CAN Pack2/6
  MeaModule7/1 -> CAN Pack2/7
  MeaModule8/1 -> CAN Pack2/8
  MeaModule6/1 -> CAN Pack2/9
  CAN Pack2/1 -> CANPackMessage2/1
  CAN Pack1/1 -> CANPackMessage1/1
  MeaModule9/1 -> WAIT_START/1
  Bus Selector/3 -> BMS_Wo/1  "<BMS_Wo>"
  [H1] -> CAN Pack1/1
  [L1] -> CAN Pack1/2
  [H2] -> CAN Pack2/1
  [L2] -> CAN Pack2/2
  Bus Selector4/1 -> CAN Pack2/4  "<Main_Contactor>"
  Bus Selector1/1 -> CAN Pack1/4  "<Main_Contactor>"
  Bus Selector3/4 -> CAN Pack5/13  "<Pedal_trav>"
  Bus Selector5/7 -> CAN Pack5/11  "<Inertia_Swich>"
  Bus Selector3/5 -> CAN Pack5/15  "<Speed>"
  Bus Selector5/8 -> CAN Pack5/12  "<LMCU>"
  CANPackMessage5/1 -> CANTransmit5/1
  Bus Selector5/4 -> CAN Pack5/8  "<Emer_Stop>"
  Constant1/1 -> CAN Pack5/7
  Bus Selector3/1 -> CAN Pack5/1  "<SteeringAngle>"
  Bus Selector5/9 -> CAN Pack5/14  "<RMCU>"
  Bus Selector3/3 -> CAN Pack5/6  "<MODE>"
  Bus Selector5/6 -> CAN Pack5/10  "<IMD_Safe>"
  Bus Selector5/3 -> CAN Pack5/4  "<Brake_Overtr_Switch>"
  Bus Selector5/5 -> CAN Pack5/9  "<HVD>"
  CANTransmit5/1 -> MeaModule1/1
  Bus Selector5/1 -> CAN Pack5/2  "<BMS_Safe>"
  MeaModule1/1 -> Terminator9/1
  CAN Pack5/1 -> CANPackMessage5/1
  Bus Selector5/2 -> CAN Pack5/3  "<BSPD_Safe>"
  Bus Selector3/2 -> CAN Pack5/5  "<Brake>"
  Bus Selector9/4 -> [L2]  "<DC_BusVoltL2>"
  Bus Selector9/1 -> [H1]  "<DC_BusVoltH1>"
  Bus Selector9/2 -> [L1]  "<DC_BusVoltL1>"
  In2/1 -> Bus Selector5/1, Bus Selector9/1
  Bus Selector9/3 -> [H2]  "<DC_BusVoltH2>"

== system Demo919/Function-Call Subsystem/Function-Call Subsystem ==
  In1 : Inport
  ID : Inport  Port=2
  Msg : Inport  Port=3
  function : TriggerPort  TriggerType=function-call  VariantControl=Variant
  Enabled Subsystem : Subsystem  TreatAsAtomicUnit=on
  Bat_Voltage_LSB : Outport
  Bat_Current_MSB : Outport  Port=2
  BatAlmLv : Outport  Port=3
  BatLife : Outport  Port=4
  BatSoc : Outport  Port=5
  BatSoh : Outport  Port=6
  BatState : Outport  Port=7
  Bat_Current_LSB : Outport  Port=8
  Bat_Voltage_MSB : Outport  Port=9
  wires:
  In1/1 -> Enabled Subsystem/Enable
  ID/1 -> Enabled Subsystem/1(In1)
  Msg/1 -> Enabled Subsystem/2(In2)
  Enabled Subsystem/1("Bat_Voltage_LSB ") -> Bat_Voltage_LSB/1
  Enabled Subsystem/2(Bat_Current_MSB) -> Bat_Current_MSB/1
  Enabled Subsystem/3("BatAlmLv ") -> BatAlmLv/1
  Enabled Subsystem/4(BatLife) -> BatLife/1
  Enabled Subsystem/5(BatSoc) -> BatSoc/1
  Enabled Subsystem/6(BatSoh) -> BatSoh/1
  Enabled Subsystem/7(BatState) -> BatState/1
  Enabled Subsystem/8(Bat_Current_LSB) -> Bat_Current_LSB/1
  Enabled Subsystem/9("Bat_Voltage_MSB ") -> Bat_Voltage_MSB/1

== system Demo919/Function-Call Subsystem/Function-Call Subsystem1 ==
  In1 : Inport
  ID : Inport  Port=2
  Msg : Inport  Port=3
  function : TriggerPort  TriggerType=function-call  VariantControl=Variant
  Enabled Subsystem : Subsystem  TreatAsAtomicUnit=on
  Re_Mot_SpeedH1 : Outport
  Re_Mot_SpeedL1 : Outport  Port=2
  Re_Mot_TorqueH1 : Outport  Port=3
  Re_Mot_TorqueL1 : Outport  Port=4
  MCU1_rdy : Outport  Port=5
  wires:
  Msg/1 -> Enabled Subsystem/2(In2)
  ID/1 -> Enabled Subsystem/1(In1)
  In1/1 -> Enabled Subsystem/Enable
  Enabled Subsystem/1(Pe_Mot_SpeedH1) -> Re_Mot_SpeedH1/1
  Enabled Subsystem/2(Re_MotSpeedL1) -> Re_Mot_SpeedL1/1
  Enabled Subsystem/3(Re_Mot_TorqueH1) -> Re_Mot_TorqueH1/1
  Enabled Subsystem/4(Re_MotTorqueL1) -> Re_Mot_TorqueL1/1
  Enabled Subsystem/5(MCU1State1) -> MCU1_rdy/1

== system Demo919/Function-Call Subsystem/Function-Call Subsystem2 ==
  In1 : Inport
  ID : Inport  Port=2
  Msg : Inport  Port=3
  function : TriggerPort  TriggerType=function-call  VariantControl=Variant
  Enabled Subsystem : Subsystem  TreatAsAtomicUnit=on
  PitchH : Outport
  PitchL : Outport  Port=2
  RollH : Outport  Port=3
  RollL : Outport  Port=4
  wires:
  In1/1 -> Enabled Subsystem/Enable
  ID/1 -> Enabled Subsystem/1(In1)
  Msg/1 -> Enabled Subsystem/2(In2)
  Enabled Subsystem/1(PitchH) -> PitchH/1
  Enabled Subsystem/3(RollH) -> RollH/1
  Enabled Subsystem/4(RollL) -> RollL/1
  Enabled Subsystem/2(PitchL) -> PitchL/1

== system Demo919/Function-Call Subsystem/Function-Call Subsystem3 ==
  In1 : Inport
  ID : Inport  Port=2
  Msg : Inport  Port=3
  function : TriggerPort  TriggerType=function-call  VariantControl=Variant
  Enabled Subsystem : Subsystem  TreatAsAtomicUnit=on
  Re_Mot_SpeedH2 : Outport
  Re_Mot_SpeedL2 : Outport  Port=2
  Re_Mot_TorqueH2 : Outport  Port=3
  Re_Mot_TorqueL2 : Outport  Port=4
  MCU2_rdy : Outport  Port=5
  wires:
  Msg/1 -> Enabled Subsystem/2(In2)
  ID/1 -> Enabled Subsystem/1(In1)
  In1/1 -> Enabled Subsystem/Enable
  Enabled Subsystem/1(Re_Mot_SpeedH2) -> Re_Mot_SpeedH2/1
  Enabled Subsystem/2(Re_Mot_SpeedL2) -> Re_Mot_SpeedL2/1
  Enabled Subsystem/3(Re_Mot_TorqueH2) -> Re_Mot_TorqueH2/1
  Enabled Subsystem/4(Re_Mot_TorqueL2) -> Re_Mot_TorqueL2/1
  Enabled Subsystem/5(MCU2State1) -> MCU2_rdy/1

== system Demo919/Function-Call Subsystem/Function-Call Subsystem4 ==
  In1 : Inport
  ID : Inport  Port=2
  Msg : Inport  Port=3
  function : TriggerPort  TriggerType=function-call  VariantControl=Variant
  Enabled Subsystem : Subsystem  TreatAsAtomicUnit=on
  MotControllerTem1 : Outport
  Mot_Tem1 : Outport  Port=2
  DC_BusVoltH1 : Outport  Port=3
  DC_BusVoltL1 : Outport  Port=4
  DC_Bus_CurrH1 : Outport  Port=5
  DC_Bus_CurrL1 : Outport  Port=6
  wires:
  In1/1 -> Enabled Subsystem/Enable
  ID/1 -> Enabled Subsystem/1(In1)
  Msg/1 -> Enabled Subsystem/2(In2)
  Enabled Subsystem/1(MotControllerTem1) -> MotControllerTem1/1
  Enabled Subsystem/2(Mot_Tem1) -> Mot_Tem1/1
  Enabled Subsystem/3(DC_Bus_VoltH1) -> DC_BusVoltH1/1
  Enabled Subsystem/4(DC_Bus_VoltL1) -> DC_BusVoltL1/1
  Enabled Subsystem/5(DC_Bus_CurrH1) -> DC_Bus_CurrH1/1
  Enabled Subsystem/6(DC_Bus_CurrL1) -> DC_Bus_CurrL1/1

== system Demo919/Function-Call Subsystem/Function-Call Subsystem6 ==
  In1 : Inport
  ID : Inport  Port=2
  Msg : Inport  Port=3
  function : TriggerPort  TriggerType=function-call  VariantControl=Variant
  Enabled Subsystem : Subsystem  TreatAsAtomicUnit=on
  Dash_Key : Outport
  wires:
  In1/1 -> Enabled Subsystem/Enable
  ID/1 -> Enabled Subsystem/1(In1)
  Msg/1 -> Enabled Subsystem/2(In2)
  Enabled Subsystem/1(Out1) -> Dash_Key/1

== system Demo919/Function-Call Subsystem/Function-Call Subsystem7 ==
  In1 : Inport
  ID : Inport  Port=2
  Msg : Inport  Port=3
  function : TriggerPort  TriggerType=function-call  VariantControl=Variant
  Enabled Subsystem : Subsystem  TreatAsAtomicUnit=on
  AxH : Outport
  AxL : Outport  Port=2
  AyH : Outport  Port=3
  AyL : Outport  Port=4
  AzH : Outport  Port=5
  AzL : Outport  Port=6
  YawH : Outport  Port=7
  YawL : Outport  Port=8
  wires:
  In1/1 -> Enabled Subsystem/Enable
  ID/1 -> Enabled Subsystem/1(In1)
  Msg/1 -> Enabled Subsystem/2(In2)
  Enabled Subsystem/1(AxH) -> AxH/1
  Enabled Subsystem/3(AyH) -> AyH/1
  Enabled Subsystem/4(AyL) -> AyL/1
  Enabled Subsystem/5(AzH) -> AzH/1
  Enabled Subsystem/6(AzL) -> AzL/1
  Enabled Subsystem/7(YawH) -> YawH/1
  Enabled Subsystem/8(YawL) -> YawL/1
  Enabled Subsystem/2(AXL) -> AxL/1

== system Demo919/Function-Call Subsystem/Function-Call Subsystem8 ==
  In1 : Inport
  ID : Inport  Port=2
  Msg : Inport  Port=3
  function : TriggerPort  TriggerType=function-call  VariantControl=Variant
  Enabled Subsystem : Subsystem  TreatAsAtomicUnit=on
  MotControllerTem2 : Outport
  Mot_Tem2 : Outport  Port=2
  DC_BusVoltH2 : Outport  Port=3
  DC_BusVoltL2 : Outport  Port=4
  DC_Bus_CurrH2 : Outport  Port=5
  "DC_Bus_CurrL2 " : Outport  Port=6
  wires:
  In1/1 -> Enabled Subsystem/Enable
  ID/1 -> Enabled Subsystem/1(In1)
  Msg/1 -> Enabled Subsystem/2(In2)
  Enabled Subsystem/1(MotControllerTem2) -> MotControllerTem2/1
  Enabled Subsystem/2(Mot_Tem2) -> Mot_Tem2/1
  Enabled Subsystem/4(DC_BusVoltL2) -> DC_BusVoltL2/1
  Enabled Subsystem/3(DC_BusVoltH2) -> DC_BusVoltH2/1
  Enabled Subsystem/5(DC_Bus_CurrH1) -> DC_Bus_CurrH2/1
  Enabled Subsystem/6(DC_Bus_CurrL1) -> "DC_Bus_CurrL2 "/1

== system Demo919/Function-Call Subsystem1/Pump ==
  Mot_Tem1 : Inport
  Mot_Tem2 : Inport  Port=2
  1-D Lookup Table1 : Lookup_n-D  NumberOfTableDimensions=1  BreakpointsForDimension1=[50 60 70 80 90 100]  BreakpointsForDimension1DataTypeStr=uint16  Table=[0 1000 2000 3000 4000 5000]  TableDataTypeStr=uint16  IntermediateResultsDataTypeStr=uint16  ExtrapMethod=Clip  InternalRulePriority=Speed  OutDataTypeStr=uint16  RndMeth=Simplest  FractionDataTypeStr=double  InputSameDT=on
  1-D Lookup Table3 : Lookup_n-D  NumberOfTableDimensions=1  BreakpointsForDimension1=[50 60 70 80 90 100]  BreakpointsForDimension1DataTypeStr=uint16  Table=PUMP  TableDataTypeStr=uint16  IntermediateResultsDataTypeStr=uint16  ExtrapMethod=Clip  InternalRulePriority=Speed  OutDataTypeStr=uint16  RndMeth=Simplest  FractionDataTypeStr=double  InputSameDT=on
  Add : Sum  Inputs=+-
  Add1 : Sum  Inputs=+-
  Constant : Constant  Value=0  OutDataTypeStr=uint16
  Constant1 : Constant  Value=0  OutDataTypeStr=uint16
  Constant2 : Constant  Value=50
  Constant3 : Constant  Value=50
  Constant4 : Constant  Value=5000  OutDataTypeStr=uint16
  Constant5 : Constant  Value=5000  OutDataTypeStr=uint16
  MeaModule : ec5744lib/RapidECU_U3/07Calibration/MeaModule  signal=PumpL
      settings: SourceProductName=ECUCoder for MPC5744
  MeaModule1 : ec5744lib/RapidECU_U3/07Calibration/MeaModule  signal=PumpR
      settings: SourceProductName=ECUCoder for MPC5744
  MeaModule2 : ec5744lib/RapidECU_U3/07Calibration/MeaModule  signal=Mot_Tem1
      settings: SourceProductName=ECUCoder for MPC5744
  MeaModule3 : ec5744lib/RapidECU_U3/07Calibration/MeaModule  signal=Mot_Tem2
      settings: SourceProductName=ECUCoder for MPC5744
  Switch : Switch  Criteria=u2 > Threshold  Threshold=50
  Switch1 : Switch  Criteria=u2 > Threshold  Threshold=50
  Terminator : Terminator
  Terminator1 : Terminator
  Pump_Sp1 : Outport
  Pump_Sp2 : Outport  Port=2
  wires:
  Mot_Tem1/1 -> Add/1
  Mot_Tem2/1 -> Add1/1
  MeaModule2/1 -> Switch/1, Switch/2  "Mot_Tem2"
  Switch/1 -> 1-D Lookup Table1/1
  Constant/1 -> Switch/3
  Constant1/1 -> Switch1/3
  Switch1/1 -> 1-D Lookup Table3/1
  MeaModule3/1 -> Switch1/2, Switch1/1  "Mot_Tem2"
  Add/1 -> MeaModule2/1
  Add1/1 -> MeaModule3/1
  Constant2/1 -> Add/2
  Constant3/1 -> Add1/2
  1-D Lookup Table3/1 -> MeaModule1/1
  1-D Lookup Table1/1 -> MeaModule/1
  MeaModule/1 -> Terminator/1
  MeaModule1/1 -> Terminator1/1
  Constant5/1 -> Pump_Sp2/1
  Constant4/1 -> Pump_Sp1/1
